simulink model "Tankmodell_Schlosser_Lack_oh"  (R2015a)
settings: Solver=FixedStepDiscrete  SolverMode=SingleTasking  StartTime=0.0  StopTime=10.0  FixedStep=1e-3  RelTol=1e-3
undefined symbols (not defined in the file or in its folder): Ended, Single
libraries: mbed_spi_max11300 x5, mbed_lib x4, mbed_lib_lack x2, simulink x2
settings Model: Creator=svenl  LastModifiedBy=oh
settings OptimizationCC: OptimizeModelRefInitCode=on  LifeSpan=1
settings HardwareCC: ProdLargestAtomicInteger=Long  ProdLargestAtomicFloat=Double  ProdEndianess=LittleEndian  ProdHWDeviceType=ARM Compatible->ARM Cortex
settings RTWCC: SystemTargetFile=mbed.tlc  TemplateMakefile=mbed.tmf  Description=Mbed Target (Embedded Target)  TargetLang=C++
settings CodeAppCC: IgnoreCustomStorageClasses=off
settings STFCustomTargetCC: CombineOutputUpdateFcns=on  SupportContinuousTime=off  SupportVariableSizeSignals=off  SystemTargetFile=mbed.tlc
settings ERTTargetCC: SupportContinuousTime=off  SupportVariableSizeSignals=off  ERTCustomFileTemplate=mbed_file_process.tlc

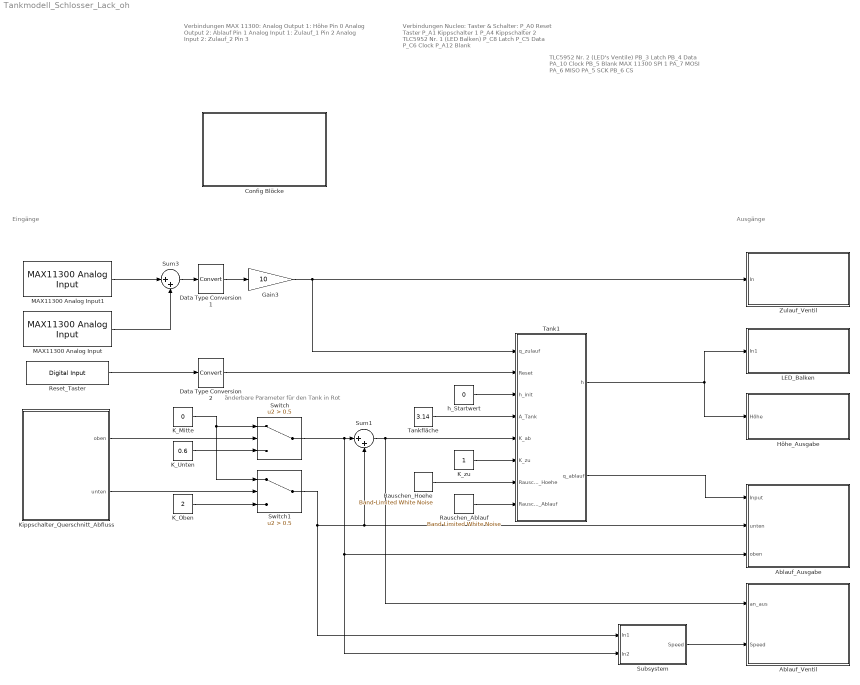
== system Tankmodell_Schlosser_Lack_oh ==
  note: Ausgänge
  note: änderbare Parameter für den Tank in Rot
  note: TLC5952 Nr. 2 (LED's Ventile)
      | PB_3 Latch
      | PB_4 Data
      | PA_10 Clock
      | PB_5 Blank
      |
      | MAX 11300 SPI 1
      | PA_7 MOSI
      | PA_6 MISO
      | PA_5 SCK
      | PB_6 CS
  note: Verbindungen Nucleo:
      |
      | Taster & Schalter:
      | P_A0 Reset Taster
      | P_A1 Kippschalter 1
      | P_A4 Kippschalter 2
      |
      | TLC5952 Nr. 1 (LED Balken)
      | P_C8 Latch
      | P_C5 Data
      | P_C6 Clock
      | P_A12 Blank
  note: Verbindungen MAX 11300:
      |
      | Analog Output 1: Höhe Pin 0
      | Analog Output 2: Ablauf Pin 1
      | Analog Input 1: Zulauf_1 Pin 2
      | Analog Input 2: Zulauf_2 Pin 3
  note: Eingänge
  Ablauf_Ausgabe : Subsystem
  Ablauf_Ventil : Subsystem
  Config Blöcke : Subsystem
  Data Type Conversion1 : DataTypeConversion
  Data Type Conversion2 : DataTypeConversion
  Gain3 : Gain  Gain=10
  Höhe_Ausgabe : Subsystem
  K_Mitte : Constant  Value=0
  K_Oben : Constant  Value=2
  K_Unten : Constant  Value=0.6
  K_zu : Constant
  Kippschalter_Querschnitt_Abfluss : Subsystem
  LED_Balken : Subsystem
  MAX11300 Analog Input : mbed_spi_max11300/MAX11300 Analog Input  CsPort=B  CsPin=6  InputType=Single-Ended  Mode=relative  PosPin=2  NegPin=0  Power=1  Range=0 to +10  Ref=Internal (2.5 V)
  MAX11300 Analog Input1 : mbed_spi_max11300/MAX11300 Analog Input  CsPort=B  CsPin=6  InputType=Single-Ended  Mode=relative  PosPin=3  NegPin=0  Power=1  Range=0 to +10  Ref=Internal (2.5 V)
  Rauschen_Ablauf : simulink/Sources/Band-Limited White Noise  Cov=[0.001]*0  Ts=0.01  seed=[23341]
  Rauschen_Hoehe : simulink/Sources/Band-Limited White Noise  Cov=[0.001]*0  Ts=0.01  seed=[23341]
  Reset_Taster : mbed_lib/GPIO/Digital Input  SParameter2=A  SParameter1=0  SParameter3=PullUp  SampleTime=-1
  Subsystem : Subsystem
  Sum1 : Sum  Inputs=|++
  Sum3 : Sum  Inputs=|++
  Switch : Switch  Criteria=u2 > Threshold  Threshold=0.5
  Switch1 : Switch  Criteria=u2 > Threshold  Threshold=0.5
  Tank1 : Subsystem
  Tankfläche : Constant  Value=3.14
  Zulauf_Ventil : Subsystem
  h_Startwert : Constant  Value=0
  wires:
  K_Mitte/1 -> Switch/1, Switch1/1
  Reset_Taster/1 -> Data Type Conversion2/1
  Tankfläche/1 -> Tank1/4("A_Tank ")
  h_Startwert/1 -> Tank1/3(h_init)
  K_Oben/1 -> Switch1/3
  K_Unten/1 -> Switch/3
  Data Type Conversion2/1 -> Tank1/2("Reset ")
  Gain3/1 -> Zulauf_Ventil/1(In), Tank1/1(q_zulauf)
  Sum1/1 -> Ablauf_Ventil/1(an_aus), Tank1/5(K_ab)
  Tank1/1(h) -> LED_Balken/1(In1), Höhe_Ausgabe/1(Höhe)
  Switch1/1 -> Subsystem/1(In1), Sum1/2, Ablauf_Ausgabe/2(unten)
  Tank1/2(q_ablauf) -> Ablauf_Ausgabe/1(Input)
  Switch/1 -> Sum1/1, Subsystem/2(In2), Ablauf_Ausgabe/3(oben)
  Kippschalter_Querschnitt_Abfluss/2(unten) -> Switch1/2
  Kippschalter_Querschnitt_Abfluss/1(oben) -> Switch/2
  Data Type Conversion1/1 -> Gain3/1
  MAX11300 Analog Input1/1 -> Sum3/1
  MAX11300 Analog Input/1 -> Sum3/2
  Sum3/1 -> Data Type Conversion1/1
  K_zu/1 -> Tank1/6(K_zu)
  Rauschen_Hoehe/1 -> Tank1/7(Rauschen_Hoehe)
  Rauschen_Ablauf/1 -> Tank1/8(Rauschen_Ablauf)
  Subsystem/1(Speed) -> Ablauf_Ventil/2("Speed ")

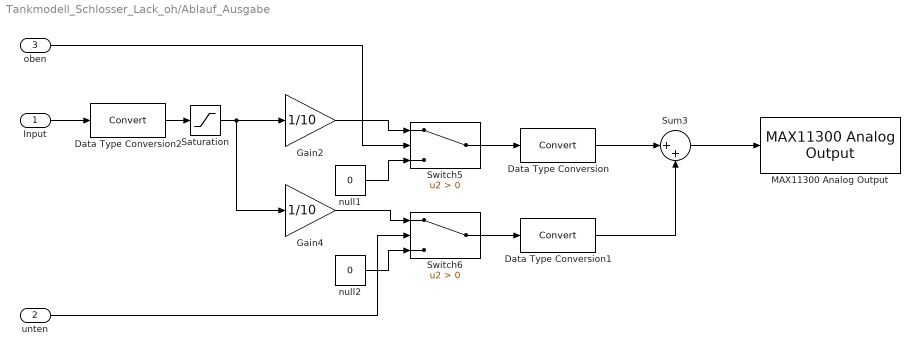
== system Tankmodell_Schlosser_Lack_oh/Ablauf_Ausgabe ==
  Input : Inport
  unten : Inport  Port=2
  oben : Inport  Port=3
  Data Type Conversion : DataTypeConversion
  Data Type Conversion1 : DataTypeConversion
  Data Type Conversion2 : DataTypeConversion
  Gain2 : Gain  Gain=1/10
  Gain4 : Gain  Gain=1/10
  MAX11300 Analog Output : mbed_spi_max11300/MAX11300 Analog Output  CsPort=B  CsPin=6  Pin=1  Mode=relative  Range=0 to +10 V
  Saturation : Saturate  UpperLimit=9.99  LowerLimit=0
  Sum3 : Sum  Inputs=|++
  Switch5 : Switch  Criteria=u2 > Threshold
  Switch6 : Switch  Criteria=u2 > Threshold
  null1 : Constant  Value=0
  null2 : Constant  Value=0
  wires:
  Saturation/1 -> Gain2/1, Gain4/1
  Data Type Conversion1/1 -> Sum3/2
  oben/1 -> Switch5/2
  Input/1 -> Data Type Conversion2/1
  unten/1 -> Switch6/2
  null1/1 -> Switch5/3
  Gain2/1 -> Switch5/1
  Switch5/1 -> Data Type Conversion/1
  Gain4/1 -> Switch6/1
  null2/1 -> Switch6/3
  Switch6/1 -> Data Type Conversion1/1
  Data Type Conversion2/1 -> Saturation/1
  Sum3/1 -> MAX11300 Analog Output/1
  Data Type Conversion/1 -> Sum3/1

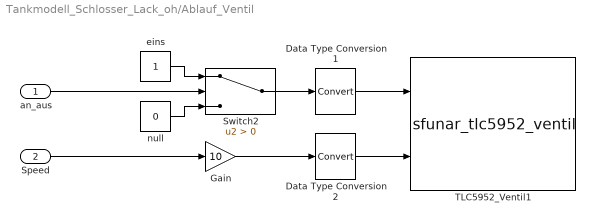
== system Tankmodell_Schlosser_Lack_oh/Ablauf_Ventil ==
  an_aus : Inport
  "Speed " : Inport  Port=2
  Data Type Conversion1 : DataTypeConversion
  Data Type Conversion2 : DataTypeConversion
  Gain : Gain  Gain=10
  Switch2 : Switch  Criteria=u2 > Threshold
  TLC5952_Ventil1 : S-Function  Priority=0  FunctionName=sfunar_tlc5952_ventil  Parameters=SampleTime, uint8(P1),uint8(P2)  mask(TLC5952 Ventil 6 LED's){P1=1, P2=1, SampleTime=-1}
      mask prompts: P1 "TLC5952 Nummer(0-5):"; P2 "Ventil Nummer(0-3):"; SampleTime "Sample time (-1 for inherited):"
      mask help: Ventil Lauflicht
      mask Help: helpview([mbed_getTargetRootPath '/doc/_build/htmlhelp/chapters/I2c_Config_en.html'])
      mask TypeOptions P1: 0 | 1 | 2 | 3 | 4
      mask TypeOptions P2: 0 | 1 | 2 | 3
      mask Display:
      | disp(['Ventil\n' 'TLC5952 Nummer ' num2str(P1-1) '\nVentil Nummer ' num2str(P2-1) ]);
      | port_label('input', 1, 'an/aus');
      | port_label('input', 2, 'Teiler Sample Time');
  eins : Constant
  null : Constant  Value=0
  wires:
  Switch2/1 -> Data Type Conversion1/1
  Data Type Conversion1/1 -> TLC5952_Ventil1/1
  an_aus/1 -> Switch2/2
  eins/1 -> Switch2/1
  null/1 -> Switch2/3
  Data Type Conversion2/1 -> TLC5952_Ventil1/2
  Gain/1 -> Data Type Conversion2/1
  "Speed "/1 -> Gain/1

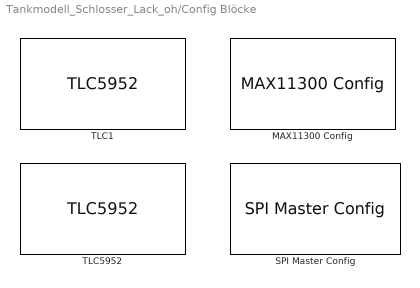
== system Tankmodell_Schlosser_Lack_oh/Config Blöcke ==
  MAX11300 Config : mbed_spi_max11300/MAX11300 Config  Priority=1  SpiPort=1  CsPort=B  CsPin=6  AdcRate=200 kSPS  DacRef=Internal (2.5 V)  TempCh0=off  TempCh1=off  TempCh2=off
  SPI Master Config : mbed_lib/SPI/SPI Master Config  Priority=0  SpiPort=1  SpiFreq=100000  MosiPort=A  MosiPin=7  MisoPort=A  MisoPin=6  SclkPort=A  SclkPin=5
  TLC1 : mbed_lib_lack/I2C/TLC5952  Priority=0  P1=C  P2=6  P3=C  P4=5  P5=C  P6=8  P7=A  P8=12  P9=10  P10=0
  TLC5952 : mbed_lib_lack/I2C/TLC5952  Priority=0  P1=A  P2=10  P3=B  P4=4  P5=B  P6=3  P7=B  P8=5  P9=15  P10=1

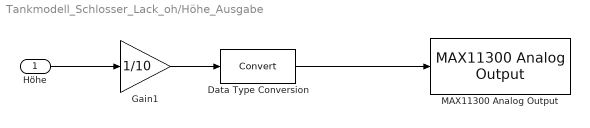
== system Tankmodell_Schlosser_Lack_oh/Höhe_Ausgabe ==
  Höhe : Inport
  Data Type Conversion : DataTypeConversion
  Gain1 : Gain  Gain=1/10
  MAX11300 Analog Output : mbed_spi_max11300/MAX11300 Analog Output  CsPort=B  CsPin=6  Pin=0  Mode=relative  Range=0 to +10 V
  wires:
  Data Type Conversion/1 -> MAX11300 Analog Output/1
  Gain1/1 -> Data Type Conversion/1
  Höhe/1 -> Gain1/1

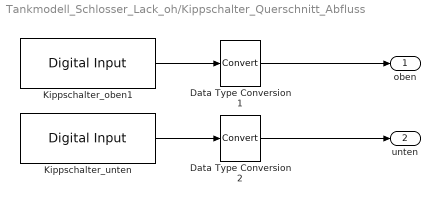
== system Tankmodell_Schlosser_Lack_oh/Kippschalter_Querschnitt_Abfluss ==
  Data Type Conversion1 : DataTypeConversion
  Data Type Conversion2 : DataTypeConversion
  Kippschalter_oben1 : mbed_lib/GPIO/Digital Input  SParameter2=A  SParameter1=1  SParameter3=PullUp  SampleTime=-1
  Kippschalter_unten : mbed_lib/GPIO/Digital Input  SParameter2=A  SParameter1=4  SParameter3=PullUp  SampleTime=-1
  oben : Outport
  unten : Outport  Port=2
  wires:
  Kippschalter_oben1/1 -> Data Type Conversion1/1
  Kippschalter_unten/1 -> Data Type Conversion2/1
  Data Type Conversion1/1 -> oben/1
  Data Type Conversion2/1 -> unten/1

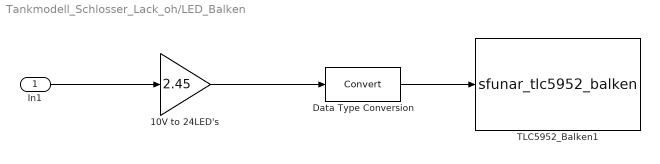
== system Tankmodell_Schlosser_Lack_oh/LED_Balken ==
  In1 : Inport
  10V to 24LED's : Gain  Gain=2.45
  Data Type Conversion : DataTypeConversion
  TLC5952_Balken1 : S-Function  Priority=0  FunctionName=sfunar_tlc5952_balken  Parameters=SampleTime,boolean(up_down) ,uint8(P1)  mask(TLC5952 Balken){P1=0, up_down=off, SampleTime=-1}
      mask prompts: P1 "TLC5952 Nummer(0-5):"; up_down "Laufrichtung (checked up/ not checked down)"; SampleTime "Sample time (-1 for inherited):"
      mask help: LED Balken mit Richtungseinstellung
      mask Help: helpview([mbed_getTargetRootPath '/doc/_build/htmlhelp/chapters/I2c_Config_en.html'])
      mask TypeOptions P1: 0 | 1 | 2 | 3 | 4
      mask Display:
      | disp(['Balken\n' 'TLC5952 Nummer ' num2str(P1)-1 ]);
      | port_label('input', 1, 'data');
  wires:
  10V to 24LED's/1 -> Data Type Conversion/1
  In1/1 -> 10V to 24LED's/1
  Data Type Conversion/1 -> TLC5952_Balken1/1

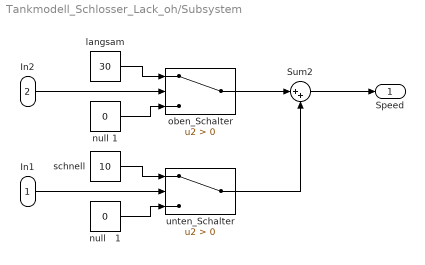
== system Tankmodell_Schlosser_Lack_oh/Subsystem ==
  In1 : Inport
  In2 : Inport  Port=2
  Sum2 : Sum  Inputs=|++
  langsam : Constant  Value=30
  null   1 : Constant  Value=0
  null 1 : Constant  Value=0
  oben_Schalter : Switch  Criteria=u2 > Threshold
  "schnell " : Constant  Value=10
  unten_Schalter : Switch  Criteria=u2 > Threshold
  Speed : Outport
  wires:
  unten_Schalter/1 -> Sum2/2
  "schnell "/1 -> unten_Schalter/1
  langsam/1 -> oben_Schalter/1
  null 1/1 -> oben_Schalter/3
  oben_Schalter/1 -> Sum2/1
  null   1/1 -> unten_Schalter/3
  Sum2/1 -> Speed/1
  In1/1 -> unten_Schalter/2
  In2/1 -> oben_Schalter/2

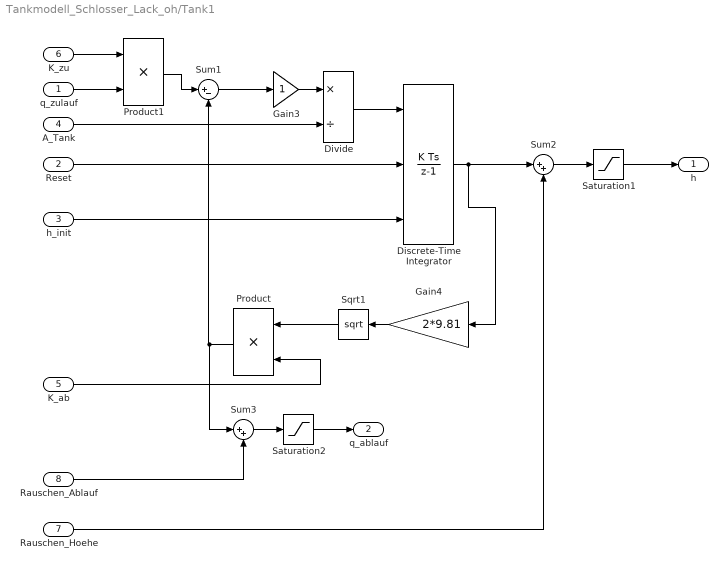
== system Tankmodell_Schlosser_Lack_oh/Tank1 ==
  q_zulauf : Inport
  "Reset " : Inport  Port=2
  h_init : Inport  Port=3
  "A_Tank " : Inport  Port=4
  K_ab : Inport  Port=5
  K_zu : Inport  Port=6
  Rauschen_Hoehe : Inport  Port=7
  Rauschen_Ablauf : Inport  Port=8
  Discrete-Time Integrator : DiscreteIntegrator  ExternalReset=falling  InitialConditionSource=external  InitialConditionSetting=State (most efficient)  SampleTime=1e-3
  Divide : Product  Inputs=*/
  Gain3 : Gain
  Gain4 : Gain  Gain=2*9.81
  Product : Product
  Product1 : Product
  Saturation1 : Saturate  UpperLimit=9.99  LowerLimit=0
  Saturation2 : Saturate  UpperLimit=9.99  LowerLimit=0
  Sqrt1 : Sqrt  SaturateOnIntegerOverflow=on
  Sum1 : Sum  Inputs=|+-
  Sum2 : Sum  Inputs=|++
  Sum3 : Sum  Inputs=|++
  h : Outport
  q_ablauf : Outport  Port=2
  wires:
  K_ab/1 -> Product/2
  Product/1 -> Sum3/1, Sum1/2
  "A_Tank "/1 -> Divide/2
  Gain3/1 -> Divide/1
  h_init/1 -> Discrete-Time Integrator/3
  "Reset "/1 -> Discrete-Time Integrator/2
  Sum1/1 -> Gain3/1
  Gain4/1 -> Sqrt1/1
  Sqrt1/1 -> Product/1
  Divide/1 -> Discrete-Time Integrator/1
  Product1/1 -> Sum1/1
  q_zulauf/1 -> Product1/2
  K_zu/1 -> Product1/1
  Discrete-Time Integrator/1 -> Gain4/1, Sum2/1
  Sum2/1 -> Saturation1/1
  Rauschen_Hoehe/1 -> Sum2/2
  Saturation1/1 -> h/1
  Saturation2/1 -> q_ablauf/1
  Sum3/1 -> Saturation2/1
  Rauschen_Ablauf/1 -> Sum3/2

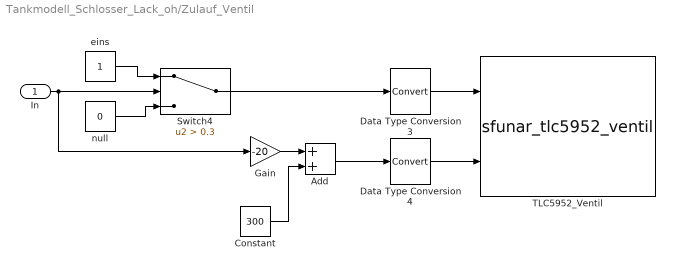
== system Tankmodell_Schlosser_Lack_oh/Zulauf_Ventil ==
  In : Inport
  Add : Sum
  Constant : Constant  Value=300
  Data Type Conversion3 : DataTypeConversion
  Data Type Conversion4 : DataTypeConversion
  Gain : Gain  Gain=-20
  Switch4 : Switch  Criteria=u2 > Threshold  Threshold=0.3
  TLC5952_Ventil : S-Function  Priority=0  FunctionName=sfunar_tlc5952_ventil  Parameters=SampleTime, uint8(P1),uint8(P2)  mask(TLC5952 Ventil 6 LED's){P1=1, P2=0, SampleTime=-1}
      mask prompts: P1 "TLC5952 Nummer(0-5):"; P2 "Ventil Nummer(0-3):"; SampleTime "Sample time (-1 for inherited):"
      mask help: Ventil Lauflicht
      mask Help: helpview([mbed_getTargetRootPath '/doc/_build/htmlhelp/chapters/I2c_Config_en.html'])
      mask TypeOptions P1: 0 | 1 | 2 | 3 | 4
      mask TypeOptions P2: 0 | 1 | 2 | 3
      mask Display:
      | disp(['Ventil\n' 'TLC5952 Nummer ' num2str(P1-1) '\nVentil Nummer ' num2str(P2-1) ]);
      | port_label('input', 1, 'an/aus');
      | port_label('input', 2, 'Teiler Sample Time');
  "eins  " : Constant
  "null " : Constant  Value=0
  wires:
  In/1 -> Gain/1, Switch4/2
  Data Type Conversion4/1 -> TLC5952_Ventil/2
  Data Type Conversion3/1 -> TLC5952_Ventil/1
  Add/1 -> Data Type Conversion4/1
  Switch4/1 -> Data Type Conversion3/1
  "eins  "/1 -> Switch4/1
  "null "/1 -> Switch4/3
  Constant/1 -> Add/2
  Gain/1 -> Add/1
